simulink model "umbral_adaptativo_base"  (R2018a)
settings: Solver=VariableStepAuto  StartTime=0.0  StopTime=0.4  MaxStep=1e-4  RelTol=1e-3
values from neighbouring files (symbols this model uses):
  tao1 = 0.002    [SimulinkInit_linea_transmision.m]
  tao2 = tao1    (= 0.002)    [SimulinkInit_linea_transmision.m]
  taod = tao1    (= 0.002)    [SimulinkInit_linea_transmision.m]
settings Model: Creator=carma  LastModifiedBy=carma

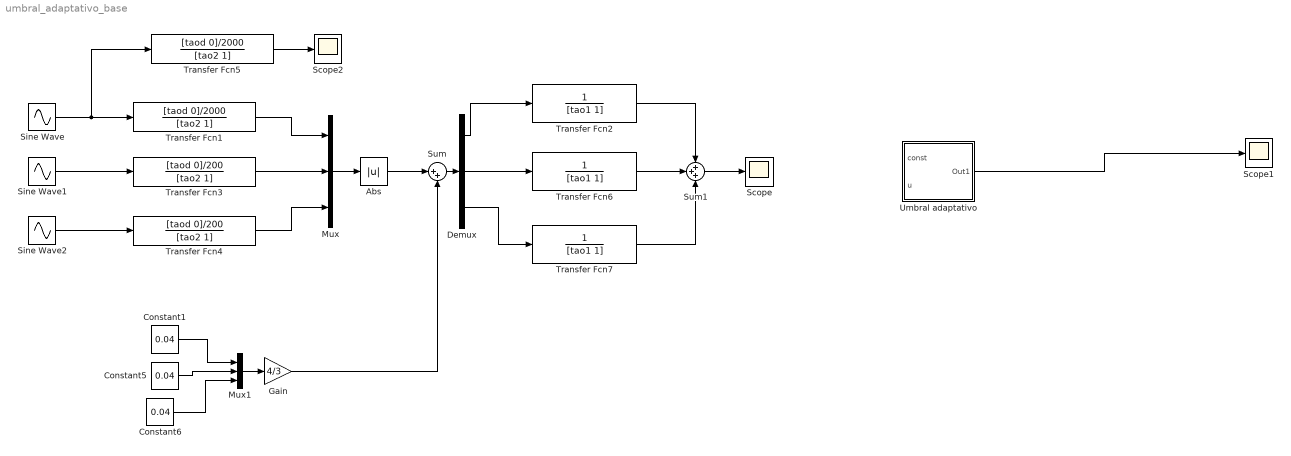
== system umbral_adaptativo_base ==
  Abs : Abs
  Constant1 : Constant  Value=0.04
  Constant5 : Constant  Value=0.04
  Constant6 : Constant  Value=0.04
  Demux : Demux  Outputs=3
  Gain : Gain  Gain=4/3
  Mux : Mux  Inputs=3
  Mux1 : Mux  Inputs=3
  Scope : Scope
  Scope1 : Scope
  Scope2 : Scope
  Sine Wave : Sin  Amplitude=2000  Frequency=2*pi*60  SampleTime=0
  Sine Wave1 : Sin  Amplitude=200  Frequency=2*pi*60  SampleTime=0
  Sine Wave2 : Sin  Amplitude=200  Frequency=2*pi*60  SampleTime=0
  Sum : Sum  Inputs=|++
  Sum1 : Sum  Inputs=3
  Transfer Fcn1 : TransferFcn  Numerator=[taod 0]/2000  Denominator=[tao2 1]
  Transfer Fcn2 : TransferFcn  Denominator=[tao1 1]
  Transfer Fcn3 : TransferFcn  Numerator=[taod 0]/200  Denominator=[tao2 1]
  Transfer Fcn4 : TransferFcn  Numerator=[taod 0]/200  Denominator=[tao2 1]
  Transfer Fcn5 : TransferFcn  Numerator=[taod 0]/2000  Denominator=[tao2 1]
  Transfer Fcn6 : TransferFcn  Denominator=[tao1 1]
  Transfer Fcn7 : TransferFcn  Denominator=[tao1 1]
  Umbral adaptativo : Subsystem
  wires:
  Mux/1 -> Abs/1
  Gain/1 -> Sum/2
  Mux1/1 -> Gain/1
  Constant1/1 -> Mux1/1
  Constant6/1 -> Mux1/3
  Constant5/1 -> Mux1/2
  Sine Wave/1 -> Transfer Fcn5/1, Transfer Fcn1/1
  Sine Wave1/1 -> Transfer Fcn3/1
  Sine Wave2/1 -> Transfer Fcn4/1
  Sum/1 -> Demux/1
  Demux/1 -> Transfer Fcn2/1
  Demux/2 -> Transfer Fcn6/1
  Demux/3 -> Transfer Fcn7/1
  Transfer Fcn1/1 -> Mux/1
  Transfer Fcn3/1 -> Mux/2
  Transfer Fcn4/1 -> Mux/3
  Transfer Fcn6/1 -> Sum1/2
  Transfer Fcn2/1 -> Sum1/1
  Transfer Fcn7/1 -> Sum1/3
  Sum1/1 -> Scope/1
  Umbral adaptativo/1(Out1) -> Scope1/1
  Transfer Fcn5/1 -> Scope2/1
  Abs/1 -> Sum/1

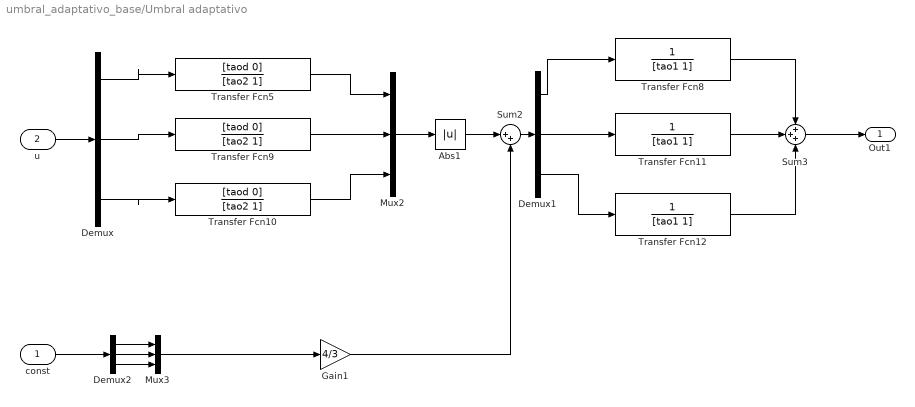
== system umbral_adaptativo_base/Umbral adaptativo ==
  const : Inport
  u : Inport  Port=2
  Abs1 : Abs
  Demux : Demux  Outputs=3
  Demux1 : Demux  Outputs=3
  Demux2 : Demux  Outputs=3
  Gain1 : Gain  Gain=4/3
  Mux2 : Mux  Inputs=3
  Mux3 : Mux  Inputs=3
  Sum2 : Sum  Inputs=|++
  Sum3 : Sum  Inputs=3
  Transfer Fcn10 : TransferFcn  Numerator=[taod 0]  Denominator=[tao2 1]
  Transfer Fcn11 : TransferFcn  Denominator=[tao1 1]
  Transfer Fcn12 : TransferFcn  Denominator=[tao1 1]
  Transfer Fcn5 : TransferFcn  Numerator=[taod 0]  Denominator=[tao2 1]
  Transfer Fcn8 : TransferFcn  Denominator=[tao1 1]
  Transfer Fcn9 : TransferFcn  Numerator=[taod 0]  Denominator=[tao2 1]
  Out1 : Outport
  wires:
  Demux1/2 -> Transfer Fcn11/1
  Sum2/1 -> Demux1/1
  Abs1/1 -> Sum2/1
  Demux1/1 -> Transfer Fcn8/1
  Gain1/1 -> Sum2/2
  Mux3/1 -> Gain1/1
  Transfer Fcn9/1 -> Mux2/2
  Transfer Fcn8/1 -> Sum3/1
  Demux1/3 -> Transfer Fcn12/1
  Mux2/1 -> Abs1/1
  Transfer Fcn5/1 -> Mux2/1
  Transfer Fcn11/1 -> Sum3/2
  Transfer Fcn12/1 -> Sum3/3
  Transfer Fcn10/1 -> Mux2/3
  Sum3/1 -> Out1/1
  Demux/2 -> Transfer Fcn9/1
  Demux/1 -> Transfer Fcn5/1
  Demux/3 -> Transfer Fcn10/1
  Demux2/1 -> Mux3/1
  Demux2/2 -> Mux3/2
  Demux2/3 -> Mux3/3
  const/1 -> Demux2/1
  u/1 -> Demux/1
